simulink model "TwoLinkRobotOL"  (R2018b)
settings: Solver=VariableStepAuto  StartTime=0.0  StopTime=5  RelTol=1e-5
libraries: ltvlib x3
settings Model: Creator=pjseiler  LastModifiedBy=jyotbuch
settings SFSimCC: SimUseLocalCustomCode=off
settings RTWCC: RTWUseLocalCustomCode=off
settings CodeAppCC: StateflowObjectComments=on

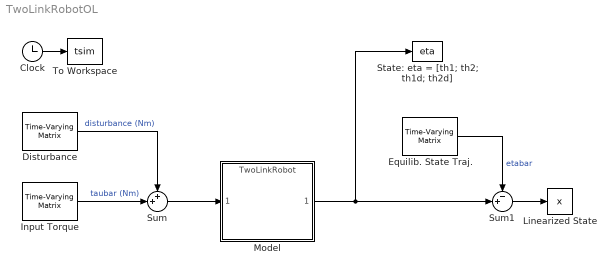
== system TwoLinkRobotOL ==
  Clock : Clock
  Disturbance : ltvlib/Time-Varying Matrix  M=d  vec1D=on
      settings: SourceProductName=Linear Time-Varying Systems Toolbox
  Equilib. State Traj. : ltvlib/Time-Varying Matrix  M=etabar  vec1D=on
      settings: SourceProductName=Linear Time-Varying Systems Toolbox
  Input Torque : ltvlib/Time-Varying Matrix  M=taubar  vec1D=on
      settings: SourceProductName=Linear Time-Varying Systems Toolbox
  Linearized State : ToWorkspace  VariableName=x  SampleTime=-1
  Model : ModelReference  ModelNameDialog=TwoLinkRobot  SimulationMode=Normal  ModelReferenceVersion=1.1
  State: eta = [th1; th2; th1d; th2d] : ToWorkspace  VariableName=eta  SampleTime=-1
  Sum : Sum  Inputs=++|
  Sum1 : Sum  Inputs=-+|
  To Workspace : ToWorkspace  VariableName=tsim  SampleTime=-1
  wires:
  Disturbance/1 -> Sum/1  "disturbance (Nm)"
  Input Torque/1 -> Sum/2  "taubar (Nm)"
  Clock/1 -> To Workspace/1
  Sum/1 -> Model/1
  Model/1 -> Sum1/2, State: eta = [th1; th2; th1d; th2d]/1
  Equilib. State Traj./1 -> Sum1/1  "etabar"
  Sum1/1 -> Linearized State/1
